simulink model "cacc_consensus_test_full_system"  (R2022b)
settings: Solver=VariableStepAuto  StartTime=0.0  StopTime=60  RelTol=1e-3
values from neighbouring files (symbols this model uses):
  A = [0 1 0; 0 0 1; 0 0 -1/tau]    [cacc_consensus_main.m]    (also in dyn_graph.m; dyn_graph_10.m; dyn_graph_10_disturb.m; fixed_graph.m)
  B = [0 0 1/tau]'    [cacc_consensus_main.m]    (also in dyn_graph.m; dyn_graph_10.m; dyn_graph_10_disturb.m; fixed_graph.m)
  C = diag([1 1 1])    [cacc_consensus_main.m]    (also in dyn_graph.m; dyn_graph_10.m; dyn_graph_10_disturb.m; fixed_graph.m)
  D = [0 0 0]'    [cacc_consensus_main.m]    (also in dyn_graph.m; dyn_graph_10.m; dyn_graph_10_disturb.m; fixed_graph.m)
  K_cacc = K_lqr    [cacc_consensus_main.m]    (also in dyn_graph.m = -K_lmi; fixed_graph.m = -K_lmi; fixed_graph_lpv.m = -K_lmi)
libraries: cstblocks x8, simulink x2
settings Model: Creator=phatdo  LastModifiedBy=phatdo
settings DataIOCC: ReturnWorkspaceOutputs=off

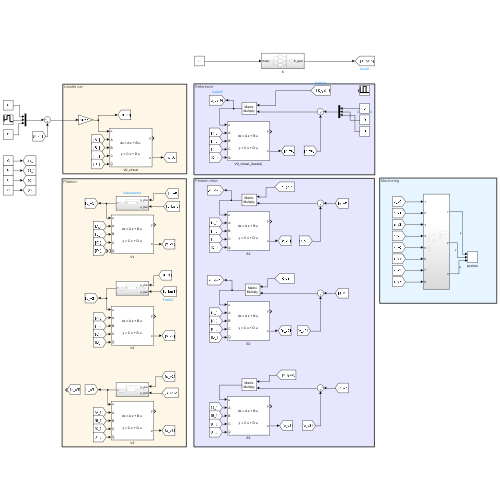
[thumbnail: Simulink's stored preview of the top-level diagram]
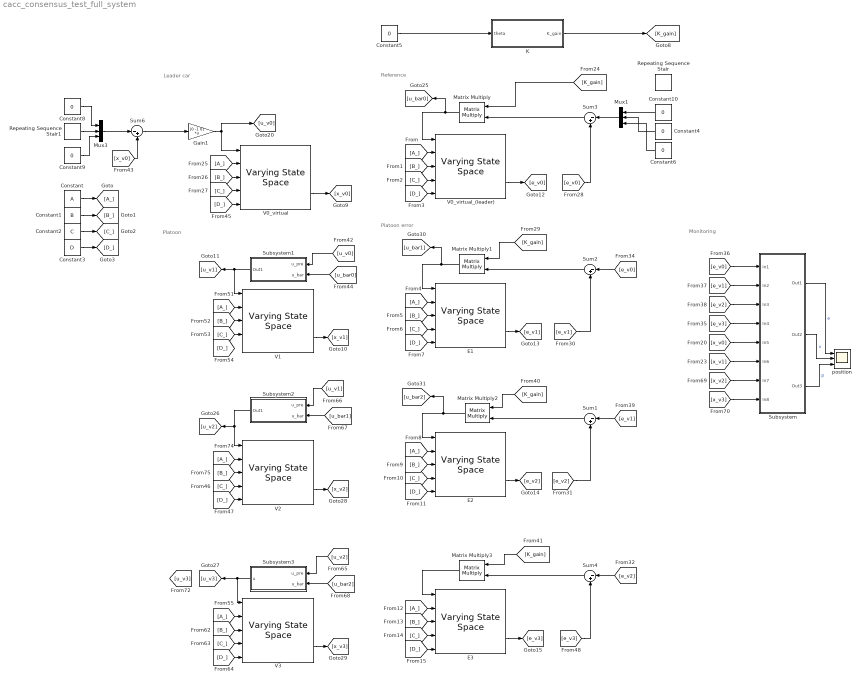
== system cacc_consensus_test_full_system ==
  note: Leader car
  note: Platoon
  note: Monitoring
  note: Reference
  note: Platoon error
  Constant : Constant  Value=A
  Constant1 : Constant  Value=B
  Constant{4..6,8..10} (6 alike) : Constant  Value=0
  Constant2 : Constant  Value=C
  Constant3 : Constant  Value=D
  E1 : cstblocks/Linear Parameter Varying/Varying State Space  x0=[0.7;0;0]  xNames=''  OutputX=on  OutputDX=off
  E2 : cstblocks/Linear Parameter Varying/Varying State Space  x0=[0.4;0;0]  xNames=''  OutputX=on  OutputDX=off
  E3 : cstblocks/Linear Parameter Varying/Varying State Space  x0=[-1 ;0 ; 0]  xNames=''  OutputX=on  OutputDX=off
  Gain1 : Gain  Gain=[0 -1 0]  Multiplication=Matrix(K*u) (u vector)
  K : Subsystem
  Matrix Multiply{,1..3} (4 alike) : Product  Multiplication=Matrix(*)
  Mux1 : Mux  Inputs=3
  Mux3 : Mux  Inputs=3
  Repeating Sequence Stair : simulink/Sources/Repeating Sequence Stair  OutValues=[0 5 0]  tsamp=20  OutMin=[]  OutMax=[]  OutDataTypeStr=double  OutputDataTypeScalingMode=double  OutDataType=fixdt(0,8)  ConRadixGroup=Best Precision: Vector-wise  OutScaling=2^-12
  Repeating Sequence Stair1 : simulink/Sources/Repeating Sequence Stair  OutValues=[20 40 10]  tsamp=20  OutMin=[]  OutMax=[]  OutDataTypeStr=double  OutputDataTypeScalingMode=double  OutDataType=fixdt(0,8)  ConRadixGroup=Best Precision: Vector-wise  OutScaling=2^-12
  Subsystem : Subsystem
  Subsystem1 : Subsystem
  Subsystem2 : Subsystem
  Subsystem3 : Subsystem
  Sum{1..4,6} (5 alike) : Sum  Inputs=|-+
  V0_virtual : cstblocks/Linear Parameter Varying/Varying State Space  x0=[0;0;0]  xNames=''  OutputX=on  OutputDX=off
  V0_virtual_(leader) : cstblocks/Linear Parameter Varying/Varying State Space  x0=[0;0;0]  xNames=''  OutputX=on  OutputDX=off
  V1 : cstblocks/Linear Parameter Varying/Varying State Space  x0=[0;0;0]  xNames=''  OutputX=on  OutputDX=off
  V2 : cstblocks/Linear Parameter Varying/Varying State Space  x0=[0;0;0]  xNames=''  OutputX=on  OutputDX=off
  V3 : cstblocks/Linear Parameter Varying/Varying State Space  x0=[0 ;0 ; 0]  xNames=''  OutputX=on  OutputDX=off
  position : Scope  NumInputPorts=3
  wires:
  Sum3/1 -> Matrix Multiply/2
  Sum2/1 -> Matrix Multiply1/2
  Sum1/1 -> Matrix Multiply2/2
  Constant2/1 -> [C_]
  Constant/1 -> [A_]
  Constant3/1 -> [D_]
  Constant1/1 -> [B_]
  [B_] -> V0_virtual_(leader)/3
  [A_] -> V0_virtual_(leader)/2
  [C_] -> V0_virtual_(leader)/4
  [D_] -> V0_virtual_(leader)/5
  [D_] -> E1/5
  [A_] -> E2/2
  [A_] -> E3/2
  [A_] -> E1/2
  [B_] -> E1/3
  [C_] -> E1/4
  [B_] -> E2/3
  [C_] -> E2/4
  [D_] -> E2/5
  [B_] -> E3/3
  [C_] -> E3/4
  [D_] -> E3/5
  Constant5/1 -> K/1(theta)
  K/1(K_gain) -> [K_gain]
  [K_gain] -> Matrix Multiply/1
  Matrix Multiply/1 -> V0_virtual_(leader)/1, [u_bar0]
  V0_virtual_(leader)/2 -> [e_v0]
  Matrix Multiply1/1 -> [u_bar1], E1/1
  [K_gain] -> Matrix Multiply1/1
  E1/2 -> [e_v1]
  [e_v0] -> Sum3/2
  [e_v1] -> Sum2/2
  Matrix Multiply2/1 -> [u_bar2], E2/1
  E2/2 -> [e_v2]
  [e_v2] -> Sum1/2
  E3/2 -> [e_v3]
  Mux1/1 -> Sum3/1
  [e_v0] -> Sum2/1
  [e_v1] -> Sum1/1
  [K_gain] -> Matrix Multiply2/1
  Matrix Multiply3/1 -> E3/1
  [K_gain] -> Matrix Multiply3/1
  [e_v3] -> Sum4/2
  Sum4/1 -> Matrix Multiply3/2
  [e_v2] -> Sum4/1
  Constant4/1 -> Mux1/2
  Constant6/1 -> Mux1/3
  Repeating Sequence Stair1/1 -> Mux3/2
  [A_] -> V1/2
  [C_] -> V1/4
  [D_] -> V0_virtual/5
  Subsystem1/1(Out1) -> V1/1, [u_v1]
  V0_virtual/2 -> [x_v0]
  [B_] -> V0_virtual/3
  [u_v0] -> Subsystem1/1(u_pre)
  [A_] -> V0_virtual/2
  [u_bar0] -> Subsystem1/2(u_bar)
  V1/2 -> [x_v1]
  Constant9/1 -> Mux3/3
  Constant8/1 -> Mux3/1
  [x_v0] -> Sum6/2
  [C_] -> V0_virtual/4
  [B_] -> V1/3
  Constant10/1 -> Mux1/1
  Sum6/1 -> Gain1/1
  [D_] -> V3/5
  V3/2 -> [x_v3]
  [A_] -> V3/2
  [B_] -> V3/3
  [u_v1] -> Subsystem2/1(u_pre)
  Subsystem2/1(Out1) -> [u_v2], V2/1
  [C_] -> V2/4
  V2/2 -> [x_v2]
  [u_bar2] -> Subsystem3/2(u_bar)
  [D_] -> V2/5
  [C_] -> V3/4
  [A_] -> V2/2
  [B_] -> V2/3
  [u_bar1] -> Subsystem2/2(u_bar)
  [u_v2] -> Subsystem3/1(u_pre)
  Subsystem3/1(u) -> V3/1, [u_v3]
  [e_v0] -> Subsystem/1(In1)
  [e_v1] -> Subsystem/2(In2)
  [e_v2] -> Subsystem/3(In3)
  [e_v3] -> Subsystem/4(In4)
  [x_v0] -> Subsystem/5(In5)
  [x_v1] -> Subsystem/6(In6)
  [x_v2] -> Subsystem/7(In7)
  [x_v3] -> Subsystem/8(In8)
  Subsystem/1(Out1) -> position/1  "e"
  Subsystem/2(Out2) -> position/2  "v"
  Subsystem/3(Out3) -> position/3  "p"
  Gain1/1 -> V0_virtual/1, [u_v0]
  Mux3/1 -> Sum6/1

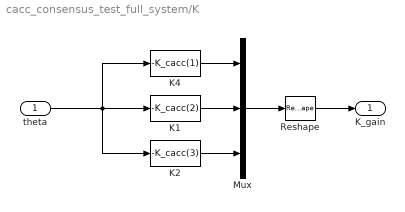
== system cacc_consensus_test_full_system/K ==
  theta : Inport
  K1 : Fcn  Expr=-K_cacc(2)
  K2 : Fcn  Expr=-K_cacc(3)
  K4 : Fcn  Expr=-K_cacc(1)
  Mux : Mux  Inputs=3
  Reshape : Reshape  OutputDimensionality=Customize  OutputDimensions=[1,3]
  K_gain : Outport
  wires:
  Mux/1 -> Reshape/1
  Reshape/1 -> K_gain/1
  K4/1 -> Mux/1
  K1/1 -> Mux/2
  K2/1 -> Mux/3
  theta/1 -> K2/1, K1/1, K4/1

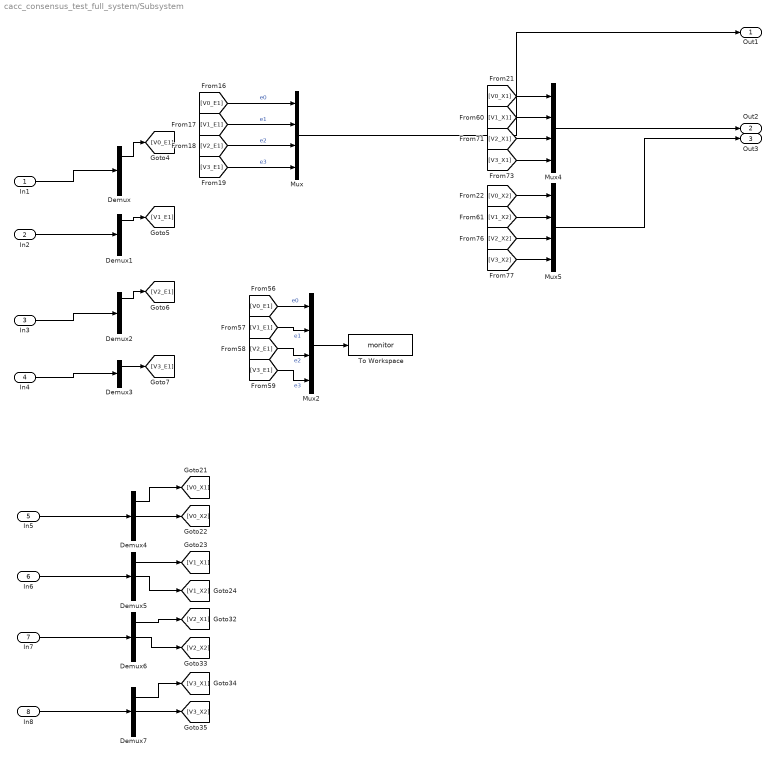
== system cacc_consensus_test_full_system/Subsystem ==
  In1 : Inport
  In2 : Inport  Port=2
  In3 : Inport  Port=3
  In4 : Inport  Port=4
  In5 : Inport  Port=5
  In6 : Inport  Port=6
  In7 : Inport  Port=7
  In8 : Inport  Port=8
  Demux{,1..7} (8 alike) : Demux  Outputs=3
  Mux{,2,4..5} (4 alike) : Mux
  To Workspace : ToWorkspace  VariableName=monitor  SaveFormat=Timeseries  SampleTime=-1
  Out1 : Outport
  Out2 : Outport  Port=2
  Out3 : Outport  Port=3
  wires:
  [V2_X1] -> Mux4/3
  Demux/1 -> [V0_E1]
  Demux2/1 -> [V2_E1]
  In2/1 -> Demux1/1
  [V2_E1] -> Mux2/3  "e2"
  [V0_X1] -> Mux4/1
  Demux1/1 -> [V1_E1]
  Demux3/1 -> [V3_E1]
  [V3_X1] -> Mux4/4
  Demux6/2 -> [V2_X2]
  Demux7/1 -> [V3_X1]
  Mux2/1 -> To Workspace/1
  Demux4/1 -> [V0_X1]
  Demux4/2 -> [V0_X2]
  In7/1 -> Demux6/1
  Demux5/2 -> [V1_X2]
  Demux6/1 -> [V2_X1]
  In4/1 -> Demux3/1
  In8/1 -> Demux7/1
  [V1_X2] -> Mux5/2
  In1/1 -> Demux/1
  [V1_E1] -> Mux2/2  "e1"
  [V0_E1] -> Mux2/1  "e0"
  Mux4/1 -> Out2/1
  Mux5/1 -> Out3/1
  [V3_X2] -> Mux5/4
  [V2_X2] -> Mux5/3
  [V0_X2] -> Mux5/1
  Demux7/2 -> [V3_X2]
  [V1_E1] -> Mux/2  "e1"
  In5/1 -> Demux4/1
  [V1_X1] -> Mux4/2
  In6/1 -> Demux5/1
  [V2_E1] -> Mux/3  "e2"
  [V3_E1] -> Mux2/4  "e3"
  [V0_E1] -> Mux/1  "e0"
  Mux/1 -> Out1/1
  [V3_E1] -> Mux/4  "e3"
  In3/1 -> Demux2/1
  Demux5/1 -> [V1_X1]

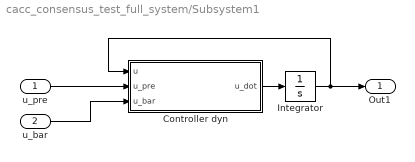
== system cacc_consensus_test_full_system/Subsystem1 ==
  u_pre : Inport
  u_bar : Inport  Port=2
  Controller dyn : MATLAB Function  TreatAsAtomicUnit=on
  Integrator : Integrator
  Out1 : Outport
  wires:
  Controller dyn/1(u_dot) -> Integrator/1
  Integrator/1 -> Controller dyn/1(u), Out1/1
  u_pre/1 -> Controller dyn/2(u_pre)
  u_bar/1 -> Controller dyn/3(u_bar)

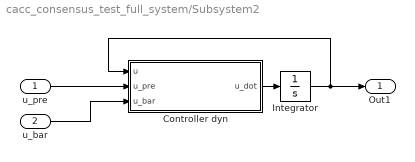
== system cacc_consensus_test_full_system/Subsystem2 ==
  u_pre : Inport
  u_bar : Inport  Port=2
  Controller dyn : MATLAB Function  TreatAsAtomicUnit=on
  Integrator : Integrator
  Out1 : Outport
  wires:
  Controller dyn/1(u_dot) -> Integrator/1
  Integrator/1 -> Controller dyn/1(u), Out1/1
  u_pre/1 -> Controller dyn/2(u_pre)
  u_bar/1 -> Controller dyn/3(u_bar)

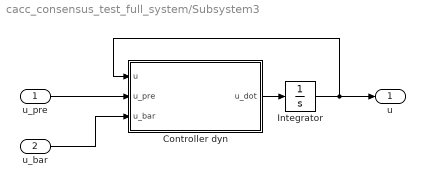
== system cacc_consensus_test_full_system/Subsystem3 ==
  u_pre : Inport
  u_bar : Inport  Port=2
  Controller dyn : MATLAB Function  TreatAsAtomicUnit=on
  Integrator : Integrator
  u : Outport
  wires:
  Controller dyn/1(u_dot) -> Integrator/1
  Integrator/1 -> Controller dyn/1(u), u/1
  u_pre/1 -> Controller dyn/2(u_pre)
  u_bar/1 -> Controller dyn/3(u_bar)

== matlab function cacc_consensus_test_full_system/Subsystem1/Controller dyn ==
  data: u input; u_dot output; u_pre input; u_bar input
function u_dot = cacc(u, u_pre, u_bar)

h = 1; % second

u_dot = -1/h * u + 1/h * (u_pre - u_bar);

end

== matlab function cacc_consensus_test_full_system/Subsystem2/Controller dyn ==
  data: u input; u_dot output; u_pre input; u_bar input
function u_dot = cacc(u, u_pre, u_bar)

h = 1; % second

u_dot = -1/h * u + 1/h * (u_pre - u_bar);

end

== matlab function cacc_consensus_test_full_system/Subsystem3/Controller dyn ==
  data: u input; u_dot output; u_pre input; u_bar input
function u_dot = cacc(u, u_pre, u_bar)

h = 1; % second

u_dot = -1/h * u + 1/h * (u_pre - u_bar);

end
